simulink model "ams"  (R2015a)
settings: Solver=ode45  StartTime=0.0  StopTime=10.0  RelTol=1e-3
settings Model: Creator=Saif Siddique  LastModifiedBy=Saif Siddique

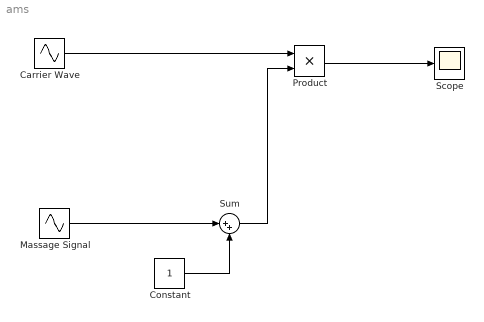
== system ams ==
  Carrier Wave : Sin  Frequency=1000  SampleTime=0.0001
  Constant : Constant
  Massage Signal : Sin  Amplitude=0.5  Frequency=10  SampleTime=0.01
  Product : Product
  Scope : Scope
  Sum : Sum  Inputs=|++
  wires:
  Constant/1 -> Sum/2
  Massage Signal/1 -> Sum/1
  Carrier Wave/1 -> Product/1
  Sum/1 -> Product/2
  Product/1 -> Scope/1
